simulink model "BrowarModel"  (R2024a)
settings: Solver=ode5  StartTime=0.0  StopTime=inf  FixedStep=0.1  RelTol=1e-3
undefined symbols (not defined in the file or in its folder): localhost, Matrikon, OI
libraries: opclib x24
(part 9 of 9)

== system BrowarModel/Mlyn browarniany/Mlyn browarniany/Zasobnik dozownika slodu/Detektory poziomu ==
  note: Detektory poziomu
  Poziom : Inport
  Pozycja sensora max (5 m) : Constant  Value=5
  Pozycja sensora min (2 m) : Constant  Value=2
  Sensor max : RelationalOperator  InputSameDT=off
  Sensor min : RelationalOperator  InputSameDT=off
  Poziom  wysoki : Outport
  Poziom niski : Outport  Port=2
  wires:
  Sensor min/1 -> Poziom niski/1
  Sensor max/1 -> Poziom  wysoki/1
  Pozycja sensora min (2 m)/1 -> Sensor min/2
  Pozycja sensora max (5 m)/1 -> Sensor max/2
  Poziom/1 -> Sensor max/1, Sensor min/1  "m"

== system BrowarModel/Mlyn browarniany/Mlyn browarniany/Zawor doplywu slodu/Zaklocenia ==
  note: Zaklocenia procesowe
  In : Inport
  Product3 : Product  InputSameDT=on  RndMeth=Zero  SaturateOnIntegerOverflow=on  OutDataTypeStr=Inherit: Same as first input
  Product4 : Product  InputSameDT=on  RndMeth=Zero  SaturateOnIntegerOverflow=on  OutDataTypeStr=Inherit: Same as first input
  Random Number : RandomNumber  Variance=0.01  Seed=4365624  SampleTime=0.1
  Transfer Fcn1 : TransferFcn  Denominator=[0.1 1]
  Out : Outport
  wires:
  [ZaklProc] -> Product3/2
  Random Number/1 -> Product3/1
  Product3/1 -> Transfer Fcn1/1
  Transfer Fcn1/1 -> Product4/2
  In/1 -> Product4/1
  Product4/1 -> Out/1

== system BrowarModel/System dozowania chmielu/System dozowania chmielu/Zasobnik/Detektory poziomu ==
  note: Detektory poziomu
  Poziom : Inport
  Pozycja sensora max (3 m) : Constant  Value=3
  Pozycja sensora min (1 m) : Constant
  Sensor max : RelationalOperator  InputSameDT=off
  Sensor min : RelationalOperator  InputSameDT=off
  Poziom  wysoki : Outport
  Poziom niski : Outport  Port=2
  wires:
  Sensor min/1 -> Poziom niski/1
  Sensor max/1 -> Poziom  wysoki/1
  Pozycja sensora min (1 m)/1 -> Sensor min/2
  Pozycja sensora max (3 m)/1 -> Sensor max/2
  Poziom/1 -> Sensor max/1, Sensor min/1  "m"

== system BrowarModel/System dozowania chmielu/System dozowania chmielu/Zawor doplywu chmielu/Zaklocenia ==
  note: Zaklocenia procesowe
  In : Inport
  Product3 : Product  InputSameDT=on  RndMeth=Zero  SaturateOnIntegerOverflow=on  OutDataTypeStr=Inherit: Same as first input
  Product4 : Product  InputSameDT=on  RndMeth=Zero  SaturateOnIntegerOverflow=on  OutDataTypeStr=Inherit: Same as first input
  Random Number : RandomNumber  Variance=0.01  Seed=4365624  SampleTime=0.1
  Transfer Fcn1 : TransferFcn  Denominator=[0.1 1]
  Out : Outport
  wires:
  [ZaklProc] -> Product3/2
  Random Number/1 -> Product3/1
  Product3/1 -> Transfer Fcn1/1
  Transfer Fcn1/1 -> Product4/2
  In/1 -> Product4/1
  Product4/1 -> Out/1

== system BrowarModel/System dozowania drozdzy/System dozowania drozdzy/Zasobnik/Detektory poziomu ==
  note: Detektory poziomu
  Poziom : Inport
  Pozycja sensora max (3 m) : Constant  Value=3
  Pozycja sensora min (1 m) : Constant
  Sensor max : RelationalOperator  InputSameDT=off
  Sensor min : RelationalOperator  InputSameDT=off
  Poziom  wysoki : Outport
  Poziom niski : Outport  Port=2
  wires:
  Sensor min/1 -> Poziom niski/1
  Sensor max/1 -> Poziom  wysoki/1
  Pozycja sensora min (1 m)/1 -> Sensor min/2
  Pozycja sensora max (3 m)/1 -> Sensor max/2
  Poziom/1 -> Sensor max/1, Sensor min/1  "m"

== system BrowarModel/System dozowania drozdzy/System dozowania drozdzy/Zawor doplywu drozdzy/Zaklocenia ==
  note: Zaklocenia procesowe
  In : Inport
  Product3 : Product  InputSameDT=on  RndMeth=Zero  SaturateOnIntegerOverflow=on  OutDataTypeStr=Inherit: Same as first input
  Product4 : Product  InputSameDT=on  RndMeth=Zero  SaturateOnIntegerOverflow=on  OutDataTypeStr=Inherit: Same as first input
  Random Number : RandomNumber  Variance=0.01  Seed=4365624  SampleTime=0.1
  Transfer Fcn1 : TransferFcn  Denominator=[0.1 1]
  Out : Outport
  wires:
  [ZaklProc] -> Product3/2
  Random Number/1 -> Product3/1
  Product3/1 -> Transfer Fcn1/1
  Transfer Fcn1/1 -> Product4/2
  In/1 -> Product4/1
  Product4/1 -> Out/1

== system BrowarModel/Kadz fermentacyjna/Kadz fermentacyjna/Kadz/Model akumulacji ciepla w zbiorniku z ciecza/Cieplo strumienia cieczy doplywajacej ==
  Temperatura strumienia cieczy : Inport
  Strumien cieczy : Inport  Port=2
  "  Dot " : DotProduct  OutDataTypeStr=Inherit: Inherit via internal rule
  Cieplo wlasciwe : Constant  Value=4189.9
  Dot : DotProduct  OutDataTypeStr=Inherit: Inherit via internal rule
  Gestosc cieczy : Gain  Gain=1000
  Sum9 : Sum  Inputs=|++
  "Zamiana C->K " : Constant  Value=273.6
  Strumien ciepla : Outport
  wires:
  Cieplo wlasciwe/1 -> Dot/1  "J/(kg*K)"
  Sum9/1 -> Dot/2  "dec K"
  "Zamiana C->K "/1 -> Sum9/2
  Dot/1 -> "  Dot "/1
  Gestosc cieczy/1 -> "  Dot "/2  "kg/s"
  Temperatura strumienia cieczy/1 -> Sum9/1
  "  Dot "/1 -> Strumien ciepla/1  "J/s"
  Strumien cieczy/1 -> Gestosc cieczy/1

== system BrowarModel/Kadz fermentacyjna/Kadz fermentacyjna/Kadz/Model akumulacji ciepla w zbiorniku z ciecza/Cieplo strumienia cieczy odplywajacej ==
  Temperatura strumienia cieczy : Inport
  Strumien cieczy : Inport  Port=2
  " Dot " : DotProduct  OutDataTypeStr=Inherit: Inherit via internal rule
  Cieplo wlasciwe : Constant  Value=4189.9
  "Dot " : DotProduct  OutDataTypeStr=Inherit: Inherit via internal rule
  Gestosc : Gain  Gain=1000
  Strumien ciepla : Outport
  wires:
  "Dot "/1 -> " Dot "/2
  Cieplo wlasciwe/1 -> "Dot "/2  "J/(kg*K)"
  Temperatura strumienia cieczy/1 -> " Dot "/1  "decK"
  Strumien cieczy/1 -> Gestosc/1  "m3/s"
  " Dot "/1 -> Strumien ciepla/1  "J/s"
  Gestosc/1 -> "Dot "/1  "kg/s"

== system BrowarModel/Kadz fermentacyjna/Kadz fermentacyjna/Kadz/Model rozkladu temperatur/Model rozkladu temperatur ==
  Poziom : Inport
  Temperatura otoczenia : Inport  Port=2
  Srednia temperatura : Inport  Port=3
  Obroty mieszadla : Inport  Port=4
  "  1/2  " : Gain  Gain=0.5
  " Dot  1" : DotProduct  OutDataTypeStr=Inherit: Inherit via internal rule
  " Gain 2" : Gain  Gain=2
  "1/2  " : Gain  Gain=0.5
  Fcn : Fcn  Expr=0.9*u(1)*(1-0.9*u(2))
  MinMax : MinMax
  Mux : Mux  Inputs=2
  Mux1 : Mux  Inputs=2
  Obroty skalowanie : Gain  Gain=1/2
  Poziom FS1 : Gain  Gain=1/2
  Sat : Saturate  UpperLimit=100  LowerLimit=0
  Sat doplyw Sat FS : Saturate  UpperLimit=1  LowerLimit=0
  Sat doplyw Sat FS1 : Saturate  UpperLimit=1  LowerLimit=0
  Saturation : Saturate  UpperLimit=100  LowerLimit=0
  Saturation1 : Saturate  UpperLimit=100  LowerLimit=0
  Sum1 : Sum  Inputs=|++
  Sum2 : Sum  Inputs=|-+
  Sum3 : Sum  Inputs=|+-
  Sum4 : Sum  Inputs=|-+
  Sum5 : Sum  Inputs=|++
  Sum7 : Sum  Inputs=|-+
  Sum8 : Sum  Inputs=|++
  Transfer Fcn : TransferFcn  Denominator=[10 1]
  Temperatura przy powierzchni : Outport
  Temperatura przy dnie : Outport  Port=2
  Gradient temperatury : Outport  Port=3
  wires:
  Srednia temperatura/1 -> Sum8/2, Sum4/2, Sum1/2, Sum2/2, Sum3/2, Sum5/2, Sum7/2
  Transfer Fcn/1 -> Sat doplyw Sat FS1/1
  Sat doplyw Sat FS1/1 -> " Dot  1"/1
  Sum4/1 -> " Dot  1"/2
  " Dot  1"/1 -> "1/2  "/1, "  1/2  "/1
  "1/2  "/1 -> Sum1/1
  "  1/2  "/1 -> Sum2/1
  Sum2/1 -> Saturation/1
  Sum1/1 -> Saturation1/1
  Saturation1/1 -> Sum3/1
  Saturation/1 -> Sum5/1
  Sum5/1 -> Mux/1
  Sum3/1 -> Mux/2
  Mux/1 -> MinMax/1
  MinMax/1 -> Sat/1
  Sat/1 -> Sum8/1, Sum7/1, " Gain 2"/1
  Temperatura otoczenia/1 -> Sum4/1
  Sum7/1 -> Temperatura przy powierzchni/1
  " Gain 2"/1 -> Gradient temperatury/1
  Sum8/1 -> Temperatura przy dnie/1
  Mux1/1 -> Fcn/1
  Poziom FS1/1 -> Mux1/1
  Sat doplyw Sat FS/1 -> Mux1/2
  Poziom/1 -> Poziom FS1/1  "m"
  Obroty mieszadla/1 -> Obroty skalowanie/1  "obr/min"
  Obroty skalowanie/1 -> Sat doplyw Sat FS/1  "FS"
  Fcn/1 -> Transfer Fcn/1

== system BrowarModel/Kadz fermentacyjna/Kadz fermentacyjna/Odplyw z kadzi/Silnik elektryczny/Stan ==
  Zalaczony : Inport
  Zdatny : Inport  Port=2
  Add : Sum  Inputs=+++
  Alarm1 : Logic  Operator=NOT  AllPortsSameDT=off
  Alarm2 : Gain  Gain=3
  Display : Display
  GUIMon : Gain
  Idle1 : Logic  AllPortsSameDT=off
  Idle2 : Logic  Operator=NOT  AllPortsSameDT=off
  Idle3 : Gain
  Running1 : Logic  AllPortsSameDT=off
  Running2 : Gain  Gain=2
  Idle : Outport
  Running : Outport  Port=2
  Alarm : Outport  Port=3
  wires:
  Running1/1 -> Running/1, Running2/1
  Idle1/1 -> Idle/1, Idle3/1
  Zalaczony/1 -> Running1/1, Idle2/1
  Zdatny/1 -> Alarm1/1, Running1/2, Idle1/2
  Alarm1/1 -> Alarm/1, Alarm2/1
  Idle2/1 -> Idle1/1
  Idle3/1 -> Add/1
  Running2/1 -> Add/2
  Alarm2/1 -> Add/3
  Add/1 -> GUIMon/1
  GUIMon/1 -> Display/1

== system BrowarModel/Kadz fermentacyjna/Kadz fermentacyjna/Odplyw z kadzi/Silnik elektryczny/Sterowanie ==
  note: Sterowanie silnika elektrycznego
  Zadane obroty : Inport
  Zalaczenie : Inport  Port=2
  Hz : Gain  Gain=45/100
  Min sterowanie : Constant  Value=5
  Relay : Relay
  Saturation [0,100] : Saturate  UpperLimit=100  LowerLimit=0
  "Sterowanie " : DotProduct  OutDataTypeStr=Inherit: Inherit via internal rule
  Sum2 : Sum  Inputs=|++
  Sterowanie : Outport
  wires:
  Relay/1 -> "Sterowanie "/1  "{0,1}"
  Saturation [0,100]/1 -> Hz/1
  Hz/1 -> Sum2/1  "Hz"
  Min sterowanie/1 -> Sum2/2  "Hz"
  Sum2/1 -> "Sterowanie "/2
  Zalaczenie/1 -> Relay/1  "{0,1}"
  "Sterowanie "/1 -> Sterowanie/1  "Hz"
  Zadane obroty/1 -> Saturation [0,100]/1  "[0,100]"

== system BrowarModel/Kadz fermentacyjna/Kadz fermentacyjna/Odplyw z kadzi/Silnik elektryczny/Sterownik ==
  PV : Inport
  SP : Inport  Port=2
  Integrator : Integrator  LimitOutput=on  UpperSaturationLimit=50  LowerSaturationLimit=0
  K : Gain
  Saturation [0,50] : Saturate  UpperLimit=50  LowerLimit=0
  Sum2 : Sum  Inputs=|+-
  Sum3 : Sum  Inputs=|++
  Ti : Gain
  CV : Outport
  wires:
  Sum2/1 -> K/1
  Integrator/1 -> Sum3/1
  K/1 -> Ti/1, Sum3/2
  Ti/1 -> Integrator/1
  PV/1 -> Sum2/2
  SP/1 -> Sum2/1
  Sum3/1 -> Saturation [0,50]/1
  Saturation [0,50]/1 -> CV/1

== system BrowarModel/Kadz fermentacyjna/Kadz fermentacyjna/Odplyw z kadzi/Silnik elektryczny/Zaklocenia ==
  note: Zaklocenia procesowe
  In : Inport
  Product3 : Product  InputSameDT=on  RndMeth=Zero  SaturateOnIntegerOverflow=on  OutDataTypeStr=Inherit: Same as first input
  Product4 : Product  InputSameDT=on  RndMeth=Zero  SaturateOnIntegerOverflow=on  OutDataTypeStr=Inherit: Same as first input
  Random Number : RandomNumber  Variance=0.05  Seed=4365624  SampleTime=0.1
  Transfer Fcn1 : TransferFcn  Denominator=[1 1]
  Transfer Fcn2 : TransferFcn  Denominator=[1 1]
  Transfer Fcn3 : TransferFcn  Denominator=[1 1]
  Out : Outport
  wires:
  [ZaklProc] -> Product3/2
  Random Number/1 -> Product3/1
  Product3/1 -> Transfer Fcn1/1
  Transfer Fcn1/1 -> Transfer Fcn2/1
  In/1 -> Product4/1
  Product4/1 -> Out/1
  Transfer Fcn2/1 -> Transfer Fcn3/1
  Transfer Fcn3/1 -> Product4/2

== system BrowarModel/Kadz filtracji/Kadz filtracji/Doplyw kadzi/Silnik elektryczny/Stan ==
  Zalaczony : Inport
  Zdatny : Inport  Port=2
  Add : Sum  Inputs=+++
  Alarm1 : Logic  Operator=NOT  AllPortsSameDT=off
  Alarm2 : Gain  Gain=3
  Display : Display
  GUIMon : Gain
  Idle1 : Logic  AllPortsSameDT=off
  Idle2 : Logic  Operator=NOT  AllPortsSameDT=off
  Idle3 : Gain
  Running1 : Logic  AllPortsSameDT=off
  Running2 : Gain  Gain=2
  Idle : Outport
  Running : Outport  Port=2
  Alarm : Outport  Port=3
  wires:
  Running1/1 -> Running/1, Running2/1
  Idle1/1 -> Idle/1, Idle3/1
  Zalaczony/1 -> Running1/1, Idle2/1
  Zdatny/1 -> Alarm1/1, Running1/2, Idle1/2
  Alarm1/1 -> Alarm/1, Alarm2/1
  Idle2/1 -> Idle1/1
  Idle3/1 -> Add/1
  Running2/1 -> Add/2
  Alarm2/1 -> Add/3
  Add/1 -> GUIMon/1
  GUIMon/1 -> Display/1

== system BrowarModel/Kadz filtracji/Kadz filtracji/Doplyw kadzi/Silnik elektryczny/Sterowanie ==
  note: Sterowanie silnika elektrycznego
  Zadane obroty : Inport
  Zalaczenie : Inport  Port=2
  Hz : Gain  Gain=45/100
  Min sterowanie : Constant  Value=5
  Relay : Relay
  Saturation [0,100] : Saturate  UpperLimit=100  LowerLimit=0
  "Sterowanie " : DotProduct  OutDataTypeStr=Inherit: Inherit via internal rule
  Sum2 : Sum  Inputs=|++
  Sterowanie : Outport
  wires:
  Relay/1 -> "Sterowanie "/1  "{0,1}"
  Saturation [0,100]/1 -> Hz/1
  Hz/1 -> Sum2/1  "Hz"
  Min sterowanie/1 -> Sum2/2  "Hz"
  Sum2/1 -> "Sterowanie "/2
  Zalaczenie/1 -> Relay/1  "{0,1}"
  "Sterowanie "/1 -> Sterowanie/1  "Hz"
  Zadane obroty/1 -> Saturation [0,100]/1  "[0,100]"

== system BrowarModel/Kadz filtracji/Kadz filtracji/Doplyw kadzi/Silnik elektryczny/Sterownik ==
  PV : Inport
  SP : Inport  Port=2
  Integrator : Integrator  LimitOutput=on  UpperSaturationLimit=50  LowerSaturationLimit=0
  K : Gain
  Saturation [0,50] : Saturate  UpperLimit=50  LowerLimit=0
  Sum2 : Sum  Inputs=|+-
  Sum3 : Sum  Inputs=|++
  Ti : Gain
  CV : Outport
  wires:
  Sum2/1 -> K/1
  Integrator/1 -> Sum3/1
  K/1 -> Ti/1, Sum3/2
  Ti/1 -> Integrator/1
  PV/1 -> Sum2/2
  SP/1 -> Sum2/1
  Sum3/1 -> Saturation [0,50]/1
  Saturation [0,50]/1 -> CV/1

== system BrowarModel/Kadz filtracji/Kadz filtracji/Doplyw kadzi/Silnik elektryczny/Zaklocenia ==
  note: Zaklocenia procesowe
  In : Inport
  Product3 : Product  InputSameDT=on  RndMeth=Zero  SaturateOnIntegerOverflow=on  OutDataTypeStr=Inherit: Same as first input
  Product4 : Product  InputSameDT=on  RndMeth=Zero  SaturateOnIntegerOverflow=on  OutDataTypeStr=Inherit: Same as first input
  Random Number : RandomNumber  Variance=0.05  Seed=4365624  SampleTime=0.1
  Transfer Fcn1 : TransferFcn  Denominator=[1 1]
  Transfer Fcn2 : TransferFcn  Denominator=[1 1]
  Transfer Fcn3 : TransferFcn  Denominator=[1 1]
  Out : Outport
  wires:
  [ZaklProc] -> Product3/2
  Random Number/1 -> Product3/1
  Product3/1 -> Transfer Fcn1/1
  Transfer Fcn1/1 -> Transfer Fcn2/1
  In/1 -> Product4/1
  Product4/1 -> Out/1
  Transfer Fcn2/1 -> Transfer Fcn3/1
  Transfer Fcn3/1 -> Product4/2

== system BrowarModel/Kadz filtracji/Kadz filtracji/Odplyw + cyrkulacja/Silnik elektryczny/Stan ==
  Zalaczony : Inport
  Zdatny : Inport  Port=2
  Add : Sum  Inputs=+++
  Alarm1 : Logic  Operator=NOT  AllPortsSameDT=off
  Alarm2 : Gain  Gain=3
  Display : Display
  GUIMon : Gain
  Idle1 : Logic  AllPortsSameDT=off
  Idle2 : Logic  Operator=NOT  AllPortsSameDT=off
  Idle3 : Gain
  Running1 : Logic  AllPortsSameDT=off
  Running2 : Gain  Gain=2
  Idle : Outport
  Running : Outport  Port=2
  Alarm : Outport  Port=3
  wires:
  Running1/1 -> Running/1, Running2/1
  Idle1/1 -> Idle/1, Idle3/1
  Zalaczony/1 -> Running1/1, Idle2/1
  Zdatny/1 -> Alarm1/1, Running1/2, Idle1/2
  Alarm1/1 -> Alarm/1, Alarm2/1
  Idle2/1 -> Idle1/1
  Idle3/1 -> Add/1
  Running2/1 -> Add/2
  Alarm2/1 -> Add/3
  Add/1 -> GUIMon/1
  GUIMon/1 -> Display/1

== system BrowarModel/Kadz filtracji/Kadz filtracji/Odplyw + cyrkulacja/Silnik elektryczny/Sterowanie ==
  note: Sterowanie silnika elektrycznego
  Zadane obroty : Inport
  Zalaczenie : Inport  Port=2
  Hz : Gain  Gain=45/100
  Min sterowanie : Constant  Value=5
  Relay : Relay
  Saturation [0,100] : Saturate  UpperLimit=100  LowerLimit=0
  "Sterowanie " : DotProduct  OutDataTypeStr=Inherit: Inherit via internal rule
  Sum2 : Sum  Inputs=|++
  Sterowanie : Outport
  wires:
  Relay/1 -> "Sterowanie "/1  "{0,1}"
  Saturation [0,100]/1 -> Hz/1
  Hz/1 -> Sum2/1  "Hz"
  Min sterowanie/1 -> Sum2/2  "Hz"
  Sum2/1 -> "Sterowanie "/2
  Zalaczenie/1 -> Relay/1  "{0,1}"
  "Sterowanie "/1 -> Sterowanie/1  "Hz"
  Zadane obroty/1 -> Saturation [0,100]/1  "[0,100]"

== system BrowarModel/Kadz filtracji/Kadz filtracji/Odplyw + cyrkulacja/Silnik elektryczny/Sterownik ==
  PV : Inport
  SP : Inport  Port=2
  Integrator : Integrator  LimitOutput=on  UpperSaturationLimit=50  LowerSaturationLimit=0
  K : Gain
  Saturation [0,50] : Saturate  UpperLimit=50  LowerLimit=0
  Sum2 : Sum  Inputs=|+-
  Sum3 : Sum  Inputs=|++
  Ti : Gain
  CV : Outport
  wires:
  Sum2/1 -> K/1
  Integrator/1 -> Sum3/1
  K/1 -> Ti/1, Sum3/2
  Ti/1 -> Integrator/1
  PV/1 -> Sum2/2
  SP/1 -> Sum2/1
  Sum3/1 -> Saturation [0,50]/1
  Saturation [0,50]/1 -> CV/1

== system BrowarModel/Kadz filtracji/Kadz filtracji/Odplyw + cyrkulacja/Silnik elektryczny/Zaklocenia ==
  note: Zaklocenia procesowe
  In : Inport
  Product3 : Product  InputSameDT=on  RndMeth=Zero  SaturateOnIntegerOverflow=on  OutDataTypeStr=Inherit: Same as first input
  Product4 : Product  InputSameDT=on  RndMeth=Zero  SaturateOnIntegerOverflow=on  OutDataTypeStr=Inherit: Same as first input
  Random Number : RandomNumber  Variance=0.05  Seed=4365624  SampleTime=0.1
  Transfer Fcn1 : TransferFcn  Denominator=[1 1]
  Transfer Fcn2 : TransferFcn  Denominator=[1 1]
  Transfer Fcn3 : TransferFcn  Denominator=[1 1]
  Out : Outport
  wires:
  [ZaklProc] -> Product3/2
  Random Number/1 -> Product3/1
  Product3/1 -> Transfer Fcn1/1
  Transfer Fcn1/1 -> Transfer Fcn2/1
  In/1 -> Product4/1
  Product4/1 -> Out/1
  Transfer Fcn2/1 -> Transfer Fcn3/1
  Transfer Fcn3/1 -> Product4/2

== system BrowarModel/Kadz filtracji/Kadz filtracji/Zbiornik dolny/Model akumulacji ciepla w zbiorniku/Cieplo strumienia cieczy odplywajacej ==
  note: Cieplo strumienia cieczy odplywajacej
  Temperatura strumienia cieczy : Inport
  Strumien cieczy : Inport  Port=2
  " Dot " : DotProduct  OutDataTypeStr=Inherit: Inherit via internal rule
  Cieplo wlasciwe : Constant  Value=4189.9
  "Dot " : DotProduct  OutDataTypeStr=Inherit: Inherit via internal rule
  Gestosc : Gain  Gain=1000
  Strumien ciepla : Outport
  wires:
  Gestosc/1 -> "Dot "/1  "kg/s"
  " Dot "/1 -> Strumien ciepla/1  "J/s"
  Strumien cieczy/1 -> Gestosc/1  "m3/s"
  Temperatura strumienia cieczy/1 -> " Dot "/1  "decK"
  Cieplo wlasciwe/1 -> "Dot "/2  "J/(kg*K)"
  "Dot "/1 -> " Dot "/2

== system BrowarModel/Kadz filtracji/Kadz filtracji/Zbiornik dolny/Model akumulacji ciepla w zbiorniku/Cieplo strumienia doplywajacego ==
  note: Cieplo strumienia doplywajacego
  Temperatura strumienia brzeczki : Inport
  Strumien brzeczki : Inport  Port=2
  "  Dot  " : DotProduct  OutDataTypeStr=Inherit: Inherit via internal rule
  Cieplo wlasciwe brzeczki : Constant  Value=4189.9
  "Dot  " : DotProduct  OutDataTypeStr=Inherit: Inherit via internal rule
  Gestosc brzeczki : Gain  Gain=1000
  Sum3 : Sum  Inputs=|++
  "Zamiana C->K  " : Constant  Value=273.6
  Strumien ciepla : Outport
  wires:
  Strumien brzeczki/1 -> Gestosc brzeczki/1
  Temperatura strumienia brzeczki/1 -> Sum3/1
  Gestosc brzeczki/1 -> "  Dot  "/2  "kg/s"
  "Dot  "/1 -> "  Dot  "/1
  "Zamiana C->K  "/1 -> Sum3/2
  Sum3/1 -> "Dot  "/2  "dec K"
  Cieplo wlasciwe brzeczki/1 -> "Dot  "/1  "J/(kg*K)"
  "  Dot  "/1 -> Strumien ciepla/1  "J/s"

== system BrowarModel/Kadz filtracji/Kadz filtracji/Zbiornik gorny/Model akumulacji ciepla w zbiorniku/Cieplo strumienia cieczy odplywajacej ==
  note: Cieplo strumienia cieczy odplywajacej
  Temperatura strumienia cieczy : Inport
  Strumien cieczy : Inport  Port=2
  " Dot " : DotProduct  OutDataTypeStr=Inherit: Inherit via internal rule
  Cieplo wlasciwe : Constant  Value=4189.9
  "Dot " : DotProduct  OutDataTypeStr=Inherit: Inherit via internal rule
  Gestosc : Gain  Gain=1000
  Strumien ciepla : Outport
  wires:
  Gestosc/1 -> "Dot "/1  "kg/s"
  " Dot "/1 -> Strumien ciepla/1  "J/s"
  Strumien cieczy/1 -> Gestosc/1  "m3/s"
  Temperatura strumienia cieczy/1 -> " Dot "/1  "decK"
  Cieplo wlasciwe/1 -> "Dot "/2  "J/(kg*K)"
  "Dot "/1 -> " Dot "/2

== system BrowarModel/Kadz filtracji/Kadz filtracji/Zbiornik gorny/Model akumulacji ciepla w zbiorniku/Cieplo strumienia doplywajacego ==
  note: Cieplo strumienia doplywajacego
  Temperatura strumienia wody : Inport
  Strumien wody : Inport  Port=2
  Temperatura strumienia zacieru : Inport  Port=3
  Strumien zacieru : Inport  Port=4
  Temperatura strumienia brzeczki : Inport  Port=5
  Strumien brzeczki : Inport  Port=6
  "  Dot " : DotProduct  OutDataTypeStr=Inherit: Inherit via internal rule
  "  Dot 1" : DotProduct  OutDataTypeStr=Inherit: Inherit via internal rule
  "  Dot 2" : DotProduct  OutDataTypeStr=Inherit: Inherit via internal rule
  Cieplo wlasciwe brzeczki : Constant  Value=4189.9
  Cieplo wlasciwe wody : Constant  Value=4189.9
  Cieplo wlasciwe zacieru : Constant  Value=4189.9
  Dot : DotProduct  OutDataTypeStr=Inherit: Inherit via internal rule
  Dot1 : DotProduct  OutDataTypeStr=Inherit: Inherit via internal rule
  Dot2 : DotProduct  OutDataTypeStr=Inherit: Inherit via internal rule
  Gestosc brzeczki : Gain  Gain=1000
  Gestosc wody : Gain  Gain=1000
  Gestosc zacieru : Gain  Gain=1000
  Sum{1..4,9} (5 alike) : Sum  Inputs=|++
  "Zamiana C->K " : Constant  Value=273.6
  "Zamiana C->K  " : Constant  Value=273.6
  Zamiana C->K 1 : Constant  Value=273.6
  Strumien ciepla : Outport
  wires:
  Strumien wody/1 -> Gestosc wody/1
  Temperatura strumienia wody/1 -> Sum9/1
  Gestosc wody/1 -> "  Dot "/2  "kg/s"
  Dot/1 -> "  Dot "/1
  "Zamiana C->K "/1 -> Sum9/2
  Sum9/1 -> Dot/2  "dec K"
  Cieplo wlasciwe wody/1 -> Dot/1  "J/(kg*K)"
  "  Dot "/1 -> Sum1/1  "J/s"
  Sum1/1 -> Strumien ciepla/1  "J/s"
  Strumien zacieru/1 -> Gestosc zacieru/1
  Temperatura strumienia zacieru/1 -> Sum2/1
  Gestosc zacieru/1 -> "  Dot 1"/2  "kg/s"
  Dot1/1 -> "  Dot 1"/1
  Zamiana C->K 1/1 -> Sum2/2
  Sum2/1 -> Dot1/2  "dec K"
  Cieplo wlasciwe zacieru/1 -> Dot1/1  "J/(kg*K)"
  Strumien brzeczki/1 -> Gestosc brzeczki/1
  Temperatura strumienia brzeczki/1 -> Sum3/1
  Gestosc brzeczki/1 -> "  Dot 2"/2  "kg/s"
  Dot2/1 -> "  Dot 2"/1
  "Zamiana C->K  "/1 -> Sum3/2
  Sum3/1 -> Dot2/2  "dec K"
  Cieplo wlasciwe brzeczki/1 -> Dot2/1  "J/(kg*K)"
  "  Dot 1"/1 -> Sum4/1  "J/s"
  Sum4/1 -> Sum1/2
  "  Dot 2"/1 -> Sum4/2  "J/s"

== system BrowarModel/Kadz filtracji/Kadz filtracji/Zbiornik gorny/Model filtru/Booster block ==
  Fast : Constant  Value=2
  Normal : Constant
  Switch : Switch  Threshold=0.5  SaturateOnIntegerOverflow=off  InputSameDT=off
  Out : Outport
  wires:
  [TrybSym] -> Switch/2
  Fast/1 -> Switch/1
  Normal/1 -> Switch/3
  Switch/1 -> Out/1

== system BrowarModel/Kadz filtracji/Kadz filtracji/Zbiornik gorny/Silnik elektryczny/Stan ==
  Zalaczony : Inport
  Zdatny : Inport  Port=2
  Add : Sum  Inputs=+++
  Alarm1 : Logic  Operator=NOT  AllPortsSameDT=off
  Alarm2 : Gain  Gain=3
  Display : Display
  GUIMon : Gain
  Idle1 : Logic  AllPortsSameDT=off
  Idle2 : Logic  Operator=NOT  AllPortsSameDT=off
  Idle3 : Gain
  Running1 : Logic  AllPortsSameDT=off
  Running2 : Gain  Gain=2
  Idle : Outport
  Running : Outport  Port=2
  Alarm : Outport  Port=3
  wires:
  Running1/1 -> Running/1, Running2/1
  Idle1/1 -> Idle/1, Idle3/1
  Zalaczony/1 -> Running1/1, Idle2/1
  Zdatny/1 -> Alarm1/1, Running1/2, Idle1/2
  Alarm1/1 -> Alarm/1, Alarm2/1
  Idle2/1 -> Idle1/1
  Idle3/1 -> Add/1
  Running2/1 -> Add/2
  Alarm2/1 -> Add/3
  Add/1 -> GUIMon/1
  GUIMon/1 -> Display/1

== system BrowarModel/Kadz filtracji/Kadz filtracji/Zbiornik gorny/Silnik elektryczny/Sterowanie ==
  note: Sterowanie silnika elektrycznego
  Zadane obroty : Inport
  Zalaczenie : Inport  Port=2
  Hz : Gain  Gain=45/100
  Min sterowanie : Constant  Value=5
  Relay : Relay
  Saturation [0,100] : Saturate  UpperLimit=100  LowerLimit=0
  "Sterowanie " : DotProduct  OutDataTypeStr=Inherit: Inherit via internal rule
  Sum2 : Sum  Inputs=|++
  Sterowanie : Outport
  wires:
  Relay/1 -> "Sterowanie "/1  "{0,1}"
  Saturation [0,100]/1 -> Hz/1
  Hz/1 -> Sum2/1  "Hz"
  Min sterowanie/1 -> Sum2/2  "Hz"
  Sum2/1 -> "Sterowanie "/2
  Zalaczenie/1 -> Relay/1  "{0,1}"
  "Sterowanie "/1 -> Sterowanie/1  "Hz"
  Zadane obroty/1 -> Saturation [0,100]/1  "[0,100]"

== system BrowarModel/Kadz filtracji/Kadz filtracji/Zbiornik gorny/Silnik elektryczny/Sterownik ==
  PV : Inport
  SP : Inport  Port=2
  Integrator : Integrator  LimitOutput=on  UpperSaturationLimit=50  LowerSaturationLimit=0
  K : Gain
  Saturation [0,50] : Saturate  UpperLimit=50  LowerLimit=0
  Sum2 : Sum  Inputs=|+-
  Sum3 : Sum  Inputs=|++
  Ti : Gain
  CV : Outport
  wires:
  Sum2/1 -> K/1
  Integrator/1 -> Sum3/1
  K/1 -> Ti/1, Sum3/2
  Ti/1 -> Integrator/1
  PV/1 -> Sum2/2
  SP/1 -> Sum2/1
  Sum3/1 -> Saturation [0,50]/1
  Saturation [0,50]/1 -> CV/1

== system BrowarModel/Kadz filtracji/Kadz filtracji/Zbiornik gorny/Silnik elektryczny/Zaklocenia ==
  note: Zaklocenia procesowe
  In : Inport
  Product3 : Product  InputSameDT=on  RndMeth=Zero  SaturateOnIntegerOverflow=on  OutDataTypeStr=Inherit: Same as first input
  Product4 : Product  InputSameDT=on  RndMeth=Zero  SaturateOnIntegerOverflow=on  OutDataTypeStr=Inherit: Same as first input
  Random Number : RandomNumber  Variance=0.05  Seed=4365624  SampleTime=0.1
  Transfer Fcn1 : TransferFcn  Denominator=[1 1]
  Transfer Fcn2 : TransferFcn  Denominator=[1 1]
  Transfer Fcn3 : TransferFcn  Denominator=[1 1]
  Out : Outport
  wires:
  [ZaklProc] -> Product3/2
  Random Number/1 -> Product3/1
  Product3/1 -> Transfer Fcn1/1
  Transfer Fcn1/1 -> Transfer Fcn2/1
  In/1 -> Product4/1
  Product4/1 -> Out/1
  Transfer Fcn2/1 -> Transfer Fcn3/1
  Transfer Fcn3/1 -> Product4/2

== system BrowarModel/Kadz warzelna/Kadz warzelna/Model jakosci warzenia/Gotowanie /Booster block ==
  Fast : Constant  Value=12
  Normal : Constant
  Switch : Switch  Threshold=0.5  SaturateOnIntegerOverflow=off  InputSameDT=off
  Out : Outport
  wires:
  [TrybSym] -> Switch/2
  Fast/1 -> Switch/1
  Normal/1 -> Switch/3
  Switch/1 -> Out/1

== system BrowarModel/Kadz warzelna/Kadz warzelna/Odplyw z kadzi/Silnik elektryczny/Stan ==
  Zalaczony : Inport
  Zdatny : Inport  Port=2
  Add : Sum  Inputs=+++
  Alarm1 : Logic  Operator=NOT  AllPortsSameDT=off
  Alarm2 : Gain  Gain=3
  Display : Display
  GUIMon : Gain
  Idle1 : Logic  AllPortsSameDT=off
  Idle2 : Logic  Operator=NOT  AllPortsSameDT=off
  Idle3 : Gain
  Running1 : Logic  AllPortsSameDT=off
  Running2 : Gain  Gain=2
  Idle : Outport
  Running : Outport  Port=2
  Alarm : Outport  Port=3
  wires:
  Running1/1 -> Running/1, Running2/1
  Idle1/1 -> Idle/1, Idle3/1
  Zalaczony/1 -> Running1/1, Idle2/1
  Zdatny/1 -> Alarm1/1, Running1/2, Idle1/2
  Alarm1/1 -> Alarm/1, Alarm2/1
  Idle2/1 -> Idle1/1
  Idle3/1 -> Add/1
  Running2/1 -> Add/2
  Alarm2/1 -> Add/3
  Add/1 -> GUIMon/1
  GUIMon/1 -> Display/1

== system BrowarModel/Kadz warzelna/Kadz warzelna/Odplyw z kadzi/Silnik elektryczny/Sterowanie ==
  note: Sterowanie silnika elektrycznego
  Zadane obroty : Inport
  Zalaczenie : Inport  Port=2
  Hz : Gain  Gain=45/100
  Min sterowanie : Constant  Value=5
  Relay : Relay
  Saturation [0,100] : Saturate  UpperLimit=100  LowerLimit=0
  "Sterowanie " : DotProduct  OutDataTypeStr=Inherit: Inherit via internal rule
  Sum2 : Sum  Inputs=|++
  Sterowanie : Outport
  wires:
  Relay/1 -> "Sterowanie "/1  "{0,1}"
  Saturation [0,100]/1 -> Hz/1
  Hz/1 -> Sum2/1  "Hz"
  Min sterowanie/1 -> Sum2/2  "Hz"
  Sum2/1 -> "Sterowanie "/2
  Zalaczenie/1 -> Relay/1  "{0,1}"
  "Sterowanie "/1 -> Sterowanie/1  "Hz"
  Zadane obroty/1 -> Saturation [0,100]/1  "[0,100]"

== system BrowarModel/Kadz warzelna/Kadz warzelna/Odplyw z kadzi/Silnik elektryczny/Sterownik ==
  PV : Inport
  SP : Inport  Port=2
  Integrator : Integrator  LimitOutput=on  UpperSaturationLimit=50  LowerSaturationLimit=0
  K : Gain
  Saturation [0,50] : Saturate  UpperLimit=50  LowerLimit=0
  Sum2 : Sum  Inputs=|+-
  Sum3 : Sum  Inputs=|++
  Ti : Gain
  CV : Outport
  wires:
  Sum2/1 -> K/1
  Integrator/1 -> Sum3/1
  K/1 -> Ti/1, Sum3/2
  Ti/1 -> Integrator/1
  PV/1 -> Sum2/2
  SP/1 -> Sum2/1
  Sum3/1 -> Saturation [0,50]/1
  Saturation [0,50]/1 -> CV/1

== system BrowarModel/Kadz warzelna/Kadz warzelna/Odplyw z kadzi/Silnik elektryczny/Zaklocenia ==
  note: Zaklocenia procesowe
  In : Inport
  Product3 : Product  InputSameDT=on  RndMeth=Zero  SaturateOnIntegerOverflow=on  OutDataTypeStr=Inherit: Same as first input
  Product4 : Product  InputSameDT=on  RndMeth=Zero  SaturateOnIntegerOverflow=on  OutDataTypeStr=Inherit: Same as first input
  Random Number : RandomNumber  Variance=0.05  Seed=4365624  SampleTime=0.1
  Transfer Fcn1 : TransferFcn  Denominator=[1 1]
  Transfer Fcn2 : TransferFcn  Denominator=[1 1]
  Transfer Fcn3 : TransferFcn  Denominator=[1 1]
  Out : Outport
  wires:
  [ZaklProc] -> Product3/2
  Random Number/1 -> Product3/1
  Product3/1 -> Transfer Fcn1/1
  Transfer Fcn1/1 -> Transfer Fcn2/1
  In/1 -> Product4/1
  Product4/1 -> Out/1
  Transfer Fcn2/1 -> Transfer Fcn3/1
  Transfer Fcn3/1 -> Product4/2

== system BrowarModel/Kadz zacierna/Kadz zacierna/Kadz zacierna/Model akumulacji ciepla w zbiorniku z ciecza/Cieplo strumienia cieczy odplywajacej ==
  note: Cieplo strumienia cieczy odplywajacej
  Temperatura strumienia cieczy : Inport
  Strumien cieczy : Inport  Port=2
  " Dot " : DotProduct  OutDataTypeStr=Inherit: Inherit via internal rule
  Cieplo wlasciwe : Constant  Value=4189.9
  "Dot " : DotProduct  OutDataTypeStr=Inherit: Inherit via internal rule
  Gestosc : Gain  Gain=1000
  Strumien ciepla : Outport
  wires:
  Gestosc/1 -> "Dot "/1  "kg/s"
  " Dot "/1 -> Strumien ciepla/1  "J/s"
  Strumien cieczy/1 -> Gestosc/1  "m3/s"
  Temperatura strumienia cieczy/1 -> " Dot "/1  "decK"
  Cieplo wlasciwe/1 -> "Dot "/2  "J/(kg*K)"
  "Dot "/1 -> " Dot "/2

== system BrowarModel/Kadz zacierna/Kadz zacierna/Kadz zacierna/Model akumulacji ciepla w zbiorniku z ciecza/Cieplo strumienia doplywajacego ==
  note: Cieplo strumienia doplywajacego
  Temperatura strumienia wody : Inport
  Strumien wody : Inport  Port=2
  Temperatura strumienia sruty : Inport  Port=3
  Strumien sruty : Inport  Port=4
  "  Dot " : DotProduct  OutDataTypeStr=Inherit: Inherit via internal rule
  "  Dot 1" : DotProduct  OutDataTypeStr=Inherit: Inherit via internal rule
  Cieplo wlasciwe sruty : Constant  Value=4189.9
  Cieplo wlasciwe wody : Constant  Value=4189.9
  Dot : DotProduct  OutDataTypeStr=Inherit: Inherit via internal rule
  Dot1 : DotProduct  OutDataTypeStr=Inherit: Inherit via internal rule
  Gestosc sruty : Gain  Gain=1000
  Gestosc wody : Gain  Gain=1000
  Sum1 : Sum  Inputs=|++
  Sum2 : Sum  Inputs=|++
  Sum9 : Sum  Inputs=|++
  "Zamiana C->K " : Constant  Value=273.6
  Zamiana C->K 1 : Constant  Value=273.6
  Strumien ciepla : Outport
  wires:
  Strumien wody/1 -> Gestosc wody/1
  Temperatura strumienia wody/1 -> Sum9/1
  Gestosc wody/1 -> "  Dot "/2  "kg/s"
  Dot/1 -> "  Dot "/1
  "Zamiana C->K "/1 -> Sum9/2
  Sum9/1 -> Dot/2  "dec K"
  Cieplo wlasciwe wody/1 -> Dot/1  "J/(kg*K)"
  "  Dot "/1 -> Sum1/1  "J/s"
  Sum1/1 -> Strumien ciepla/1  "J/s"
  Strumien sruty/1 -> Gestosc sruty/1
  Temperatura strumienia sruty/1 -> Sum2/1
  Gestosc sruty/1 -> "  Dot 1"/2  "kg/s"
  Dot1/1 -> "  Dot 1"/1
  Zamiana C->K 1/1 -> Sum2/2
  Sum2/1 -> Dot1/2  "dec K"
  Cieplo wlasciwe sruty/1 -> Dot1/1  "J/(kg*K)"
  "  Dot 1"/1 -> Sum1/2  "J/s"

== system BrowarModel/Kadz zacierna/Kadz zacierna/Kadz zacierna/Model jakosci zacieru/Przerwa bialkowa  ==
  note: Przerwa bialkowa
  Srednia temperatura : Inport
  Jakosc mieszaniny : Inport  Port=2
  Objetosc mieszaniny : Inport  Port=3
  Odplyw : Inport  Port=4
  Obroty mieszadla : Inport  Port=5
  Booster : Product  RndMeth=Zero
  Booster block : Subsystem
  Constant : Constant  Value=0.2
  Divide : Product  Inputs=*/
  Dynamika rozkladu : Gain  Gain=1/100
  Ilosc : Integrator  LimitOutput=on  UpperSaturationLimit=48  LowerSaturationLimit=0
  Mieszadlo : DotProduct  OutDataTypeStr=Inherit: Inherit via internal rule
  Nasycenie : DotProduct  OutDataTypeStr=Inherit: Inherit via internal rule
  Odplyw srutu : DotProduct  OutDataTypeStr=Inherit: Inherit via internal rule
  Relational Operator1 : RelationalOperator  Operator=>  InputSameDT=off
  Sum : Sum  Inputs=|++
  Sum8 : Sum  Inputs=|+-
  Sum9 : Sum  Inputs=|+-
  Szybkosc reakcji : DotProduct  OutDataTypeStr=Inherit: Inherit via internal rule
  Warunki rozkladu : DotProduct  OutDataTypeStr=Inherit: Inherit via internal rule
  Wplyw mpieszadla : Gain  Gain=0.8/0.9563
  Wplyw temperatury : Lookup  InputValues=[0, 46, 49, 50, 51, 54, 100]  Table=[0, 0, 1, 1, 1 0, 0]  SaturateOnIntegerOverflow=off
  Skrobia rozpuszczona : Outport
  wires:
  Wplyw temperatury/1 -> Warunki rozkladu/2
  Ilosc/1 -> Sum8/2, Divide/1
  Szybkosc reakcji/1 -> Nasycenie/2
  Divide/1 -> Odplyw srutu/2, Relational Operator1/2, Skrobia rozpuszczona/1
  Relational Operator1/1 -> Nasycenie/1
  Sum8/1 -> Szybkosc reakcji/2
  Sum9/1 -> Ilosc/1
  Nasycenie/1 -> Sum9/1
  Odplyw srutu/1 -> Sum9/2
  Srednia temperatura/1 -> Wplyw temperatury/1
  Objetosc mieszaniny/1 -> Divide/2, Sum8/1
  Odplyw/1 -> Odplyw srutu/1
  Jakosc mieszaniny/1 -> Warunki rozkladu/1, Relational Operator1/1
  Mieszadlo/1 -> Dynamika rozkladu/1
  Warunki rozkladu/1 -> Mieszadlo/2
  Obroty mieszadla/1 -> Wplyw mpieszadla/1
  Wplyw mpieszadla/1 -> Sum/1
  Constant/1 -> Sum/2
  Sum/1 -> Mieszadlo/1
  Booster block/1(Out) -> Booster/2
  Dynamika rozkladu/1 -> Booster/1
  Booster/1 -> Szybkosc reakcji/1

== system BrowarModel/Kadz zacierna/Kadz zacierna/Kadz zacierna/Model jakosci zacieru/Przerwa dekstrynujaca ==
  note: Przerwa dekstrynujaca
  Dekstryny : Inport
  Srednia temperatura : Inport  Port=2
  Jakosc mieszaniny : Inport  Port=3
  Objetosc mieszaniny : Inport  Port=4
  Odplyw : Inport  Port=5
  Obroty mieszadla : Inport  Port=6
  Booster : Product  RndMeth=Zero
  Booster block : Subsystem
  Constant : Constant  Value=0.2
  Divide : Product  Inputs=*/
  Dynamika rozkladu : Gain  Gain=1/100
  Ilosc : Integrator  LimitOutput=on  UpperSaturationLimit=48  LowerSaturationLimit=0
  Mieszadlo : DotProduct  OutDataTypeStr=Inherit: Inherit via internal rule
  Nasycenie : DotProduct  OutDataTypeStr=Inherit: Inherit via internal rule
  Odplyw srutu : DotProduct  OutDataTypeStr=Inherit: Inherit via internal rule
  Relational Operator1 : RelationalOperator  Operator=>  InputSameDT=off
  Sum : Sum  Inputs=|++
  Sum8 : Sum  Inputs=|+-
  Sum9 : Sum  Inputs=|+-
  Szybkosc reakcji : DotProduct  OutDataTypeStr=Inherit: Inherit via internal rule
  Warunki rozkladu : DotProduct  OutDataTypeStr=Inherit: Inherit via internal rule
  Wplyw mpieszadla : Gain  Gain=0.8/0.9563
  Wplyw temperatury : Lookup  InputValues=[0, 71, 74, 75, 76, 80, 100]  Table=[0, 0, 1, 1, 1, 0, 0]  SaturateOnIntegerOverflow=off
  Maltoza : Outport
  wires:
  Wplyw temperatury/1 -> Warunki rozkladu/2
  Ilosc/1 -> Sum8/2, Divide/1
  Szybkosc reakcji/1 -> Nasycenie/2
  Divide/1 -> Odplyw srutu/2, Relational Operator1/2, Maltoza/1
  Relational Operator1/1 -> Nasycenie/1
  Sum8/1 -> Szybkosc reakcji/2
  Sum9/1 -> Ilosc/1
  Nasycenie/1 -> Sum9/1
  Odplyw srutu/1 -> Sum9/2
  Srednia temperatura/1 -> Wplyw temperatury/1
  Objetosc mieszaniny/1 -> Divide/2, Sum8/1
  Odplyw/1 -> Odplyw srutu/1
  Jakosc mieszaniny/1 -> Warunki rozkladu/1
  Dekstryny/1 -> Relational Operator1/1
  Obroty mieszadla/1 -> Wplyw mpieszadla/1
  Wplyw mpieszadla/1 -> Sum/1
  Constant/1 -> Sum/2
  Sum/1 -> Mieszadlo/1
  Booster block/1(Out) -> Booster/2
  Mieszadlo/1 -> Dynamika rozkladu/1
  Warunki rozkladu/1 -> Mieszadlo/2
  Dynamika rozkladu/1 -> Booster/1
  Booster/1 -> Szybkosc reakcji/1

== system BrowarModel/Kadz zacierna/Kadz zacierna/Kadz zacierna/Model jakosci zacieru/Przerwa maltozowa ==
  note: Przerwa maltozowa
  Skrobia rozpuszczona : Inport
  Srednia temperatura : Inport  Port=2
  Jakosc mieszaniny : Inport  Port=3
  Objetosc mieszaniny : Inport  Port=4
  Odplyw : Inport  Port=5
  Obroty mieszadla : Inport  Port=6
  Booster : Product  RndMeth=Zero
  Booster block : Subsystem
  Constant : Constant  Value=0.2
  Divide : Product  Inputs=*/
  Dynamika rozkladu : Gain  Gain=1/100
  Ilosc : Integrator  LimitOutput=on  UpperSaturationLimit=48  LowerSaturationLimit=0
  Mieszadlo : DotProduct  OutDataTypeStr=Inherit: Inherit via internal rule
  Nasycenie : DotProduct  OutDataTypeStr=Inherit: Inherit via internal rule
  Odplyw srutu : DotProduct  OutDataTypeStr=Inherit: Inherit via internal rule
  Relational Operator1 : RelationalOperator  Operator=>  InputSameDT=off
  Sum : Sum  Inputs=|++
  Sum8 : Sum  Inputs=|+-
  Sum9 : Sum  Inputs=|+-
  Szybkosc reakcji : DotProduct  OutDataTypeStr=Inherit: Inherit via internal rule
  Warunki rozkladu : DotProduct  OutDataTypeStr=Inherit: Inherit via internal rule
  Wplyw mpieszadla : Gain  Gain=0.8/0.9563
  Wplyw temperatury : Lookup  InputValues=[0, 64, 67, 68, 69, 72, 100]  Table=[0, 0, 1, 1, 1, 0, 0]  SaturateOnIntegerOverflow=off
  Dekstryny : Outport
  wires:
  Jakosc mieszaniny/1 -> Warunki rozkladu/1
  Odplyw/1 -> Odplyw srutu/1
  Objetosc mieszaniny/1 -> Sum8/1, Divide/2
  Srednia temperatura/1 -> Wplyw temperatury/1
  Odplyw srutu/1 -> Sum9/2
  Nasycenie/1 -> Sum9/1
  Sum9/1 -> Ilosc/1
  Sum8/1 -> Szybkosc reakcji/2
  Relational Operator1/1 -> Nasycenie/1
  Divide/1 -> Relational Operator1/2, Odplyw srutu/2, Dekstryny/1
  Szybkosc reakcji/1 -> Nasycenie/2
  Ilosc/1 -> Sum8/2, Divide/1
  Wplyw temperatury/1 -> Warunki rozkladu/2
  Skrobia rozpuszczona/1 -> Relational Operator1/1
  Obroty mieszadla/1 -> Wplyw mpieszadla/1
  Wplyw mpieszadla/1 -> Sum/1
  Constant/1 -> Sum/2
  Sum/1 -> Mieszadlo/1
  Warunki rozkladu/1 -> Mieszadlo/2
  Mieszadlo/1 -> Dynamika rozkladu/1
  Booster/1 -> Szybkosc reakcji/1
  Dynamika rozkladu/1 -> Booster/1
  Booster block/1(Out) -> Booster/2

== system BrowarModel/Kadz zacierna/Kadz zacierna/Kadz zacierna/Model rozkladu temperatur/Gradient temperatury ==
  note: Gradient temperatury
  Poziom : Inport
  Temperatura otoczenia : Inport  Port=2
  Srednia temperatura : Inport  Port=3
  Obroty mieszadla : Inport  Port=4
  "  1/2  " : Gain  Gain=0.5
  " Dot  1" : DotProduct  OutDataTypeStr=Inherit: Inherit via internal rule
  " Gain 2" : Gain  Gain=2
  "1/2  " : Gain  Gain=0.5
  Fcn : Fcn  Expr=0.9*u(1)*(1-0.9*u(2))
  MinMax : MinMax
  Mux : Mux  Inputs=2
  Mux1 : Mux  Inputs=2
  Obroty skalowanie : Gain  Gain=1/2
  Poziom FS1 : Gain  Gain=1/2
  Sat : Saturate  UpperLimit=100  LowerLimit=0
  Sat doplyw Sat FS : Saturate  UpperLimit=1  LowerLimit=0
  Sat doplyw Sat FS1 : Saturate  UpperLimit=1  LowerLimit=0
  Saturation : Saturate  UpperLimit=100  LowerLimit=0
  Saturation1 : Saturate  UpperLimit=100  LowerLimit=0
  Sum1 : Sum  Inputs=|++
  Sum2 : Sum  Inputs=|-+
  Sum3 : Sum  Inputs=|+-
  Sum4 : Sum  Inputs=|-+
  Sum5 : Sum  Inputs=|++
  Sum7 : Sum  Inputs=|-+
  Sum8 : Sum  Inputs=|++
  Transfer Fcn : TransferFcn  Denominator=[10 1]
  Temperatura przy powierzchni : Outport
  Temperatura przy dnie : Outport  Port=2
  Gradient temperatury : Outport  Port=3
  wires:
  Fcn/1 -> Transfer Fcn/1
  Obroty skalowanie/1 -> Sat doplyw Sat FS/1  "FS"
  Obroty mieszadla/1 -> Obroty skalowanie/1  "obr/min"
  Poziom/1 -> Poziom FS1/1  "m"
  Sat doplyw Sat FS/1 -> Mux1/2
  Poziom FS1/1 -> Mux1/1
  Mux1/1 -> Fcn/1
  Sum8/1 -> Temperatura przy dnie/1
  " Gain 2"/1 -> Gradient temperatury/1
  Sum7/1 -> Temperatura przy powierzchni/1
  Temperatura otoczenia/1 -> Sum4/1
  Sat/1 -> " Gain 2"/1, Sum7/1, Sum8/1
  MinMax/1 -> Sat/1
  Mux/1 -> MinMax/1
  Sum3/1 -> Mux/2
  Sum5/1 -> Mux/1
  Saturation/1 -> Sum5/1
  Saturation1/1 -> Sum3/1
  Sum1/1 -> Saturation1/1
  Sum2/1 -> Saturation/1
  "  1/2  "/1 -> Sum2/1
  "1/2  "/1 -> Sum1/1
  " Dot  1"/1 -> "  1/2  "/1, "1/2  "/1
  Sum4/1 -> " Dot  1"/2
  Sat doplyw Sat FS1/1 -> " Dot  1"/1
  Transfer Fcn/1 -> Sat doplyw Sat FS1/1
  Srednia temperatura/1 -> Sum7/2, Sum5/2, Sum3/2, Sum2/2, Sum1/2, Sum4/2, Sum8/2

== system BrowarModel/Mlyn browarniany/Mlyn browarniany/Dozownik mlyna/Dozownik turbinowy/Zaklocenia ==
  note: Zaklocenia procesowe
  In : Inport
  Product3 : Product  InputSameDT=on  RndMeth=Zero  SaturateOnIntegerOverflow=on  OutDataTypeStr=Inherit: Same as first input
  Product4 : Product  InputSameDT=on  RndMeth=Zero  SaturateOnIntegerOverflow=on  OutDataTypeStr=Inherit: Same as first input
  Random Number : RandomNumber  Variance=0.1  Seed=4365624  SampleTime=0.1
  Transfer Fcn1 : TransferFcn  Denominator=[1 1]
  Out : Outport
  wires:
  [ZaklProc] -> Product3/2
  Random Number/1 -> Product3/1
  Product3/1 -> Transfer Fcn1/1
  Transfer Fcn1/1 -> Product4/2
  In/1 -> Product4/1
  Product4/1 -> Out/1

== system BrowarModel/Mlyn browarniany/Mlyn browarniany/Dozownik mlyna/Silnik elektryczny/Stan ==
  Zalaczony : Inport
  Zdatny : Inport  Port=2
  Add : Sum  Inputs=+++
  Alarm1 : Logic  Operator=NOT  AllPortsSameDT=off
  Alarm2 : Gain  Gain=3
  Display : Display
  GUIMon : Gain
  Idle1 : Logic  AllPortsSameDT=off
  Idle2 : Logic  Operator=NOT  AllPortsSameDT=off
  Idle3 : Gain
  Running1 : Logic  AllPortsSameDT=off
  Running2 : Gain  Gain=2
  Idle : Outport
  Running : Outport  Port=2
  Alarm : Outport  Port=3
  wires:
  Running1/1 -> Running/1, Running2/1
  Idle1/1 -> Idle/1, Idle3/1
  Zalaczony/1 -> Running1/1, Idle2/1
  Zdatny/1 -> Alarm1/1, Running1/2, Idle1/2
  Alarm1/1 -> Alarm/1, Alarm2/1
  Idle2/1 -> Idle1/1
  Idle3/1 -> Add/1
  Running2/1 -> Add/2
  Alarm2/1 -> Add/3
  Add/1 -> GUIMon/1
  GUIMon/1 -> Display/1

== system BrowarModel/Mlyn browarniany/Mlyn browarniany/Dozownik mlyna/Silnik elektryczny/Sterowanie ==
  note: Sterowanie silnika elektrycznego
  Zadane obroty : Inport
  Zalaczenie : Inport  Port=2
  Hz : Gain  Gain=45/100
  Min sterowanie : Constant  Value=5
  Relay : Relay
  Saturation [0,100] : Saturate  UpperLimit=100  LowerLimit=0
  "Sterowanie " : DotProduct  OutDataTypeStr=Inherit: Inherit via internal rule
  Sum2 : Sum  Inputs=|++
  Sterowanie : Outport
  wires:
  Relay/1 -> "Sterowanie "/1  "{0,1}"
  Saturation [0,100]/1 -> Hz/1
  Hz/1 -> Sum2/1  "Hz"
  Min sterowanie/1 -> Sum2/2  "Hz"
  Sum2/1 -> "Sterowanie "/2
  Zalaczenie/1 -> Relay/1  "{0,1}"
  "Sterowanie "/1 -> Sterowanie/1  "Hz"
  Zadane obroty/1 -> Saturation [0,100]/1  "[0,100]"

== system BrowarModel/Mlyn browarniany/Mlyn browarniany/Dozownik mlyna/Silnik elektryczny/Sterownik ==
  PV : Inport
  SP : Inport  Port=2
  Integrator : Integrator  LimitOutput=on  UpperSaturationLimit=50  LowerSaturationLimit=0
  K : Gain
  Saturation [0,50] : Saturate  UpperLimit=50  LowerLimit=0
  Sum2 : Sum  Inputs=|+-
  Sum3 : Sum  Inputs=|++
  Ti : Gain
  CV : Outport
  wires:
  Sum2/1 -> K/1
  Integrator/1 -> Sum3/1
  K/1 -> Ti/1, Sum3/2
  Ti/1 -> Integrator/1
  PV/1 -> Sum2/2
  SP/1 -> Sum2/1
  Sum3/1 -> Saturation [0,50]/1
  Saturation [0,50]/1 -> CV/1

== system BrowarModel/Mlyn browarniany/Mlyn browarniany/Dozownik mlyna/Silnik elektryczny/Zaklocenia ==
  note: Zaklocenia procesowe
  In : Inport
  Product3 : Product  InputSameDT=on  RndMeth=Zero  SaturateOnIntegerOverflow=on  OutDataTypeStr=Inherit: Same as first input
  Product4 : Product  InputSameDT=on  RndMeth=Zero  SaturateOnIntegerOverflow=on  OutDataTypeStr=Inherit: Same as first input
  Random Number : RandomNumber  Variance=0.05  Seed=4365624  SampleTime=0.1
  Transfer Fcn1 : TransferFcn  Denominator=[1 1]
  Transfer Fcn2 : TransferFcn  Denominator=[1 1]
  Transfer Fcn3 : TransferFcn  Denominator=[1 1]
  Out : Outport
  wires:
  [ZaklProc] -> Product3/2
  Random Number/1 -> Product3/1
  Product3/1 -> Transfer Fcn1/1
  Transfer Fcn1/1 -> Transfer Fcn2/1
  In/1 -> Product4/1
  Product4/1 -> Out/1
  Transfer Fcn2/1 -> Transfer Fcn3/1
  Transfer Fcn3/1 -> Product4/2

== system BrowarModel/Mlyn browarniany/Mlyn browarniany/Walce mlyna/Komora nad walcami/Detektory poziomu ==
  note: Detektory poziomu
  Poziom : Inport
  Pozycja sensora max : Constant  Value=0.7
  Pozycja sensora min : Constant  Value=0.3
  Sensor max : RelationalOperator  InputSameDT=off
  Sensor min : RelationalOperator  InputSameDT=off
  Poziom  wysoki : Outport
  Poziom niski : Outport  Port=2
  wires:
  Sensor min/1 -> Poziom niski/1
  Sensor max/1 -> Poziom  wysoki/1
  Pozycja sensora min/1 -> Sensor min/2
  Pozycja sensora max/1 -> Sensor max/2
  Poziom/1 -> Sensor max/1, Sensor min/1  "m"

== system BrowarModel/Mlyn browarniany/Mlyn browarniany/Walce mlyna/Silnik elektryczny/Stan ==
  Zalaczony : Inport
  Zdatny : Inport  Port=2
  Add : Sum  Inputs=+++
  Alarm1 : Logic  Operator=NOT  AllPortsSameDT=off
  Alarm2 : Gain  Gain=3
  Display : Display
  GUIMon : Gain
  Idle1 : Logic  AllPortsSameDT=off
  Idle2 : Logic  Operator=NOT  AllPortsSameDT=off
  Idle3 : Gain
  Running1 : Logic  AllPortsSameDT=off
  Running2 : Gain  Gain=2
  Idle : Outport
  Running : Outport  Port=2
  Alarm : Outport  Port=3
  wires:
  Running1/1 -> Running/1, Running2/1
  Idle1/1 -> Idle/1, Idle3/1
  Zalaczony/1 -> Running1/1, Idle2/1
  Zdatny/1 -> Alarm1/1, Running1/2, Idle1/2
  Alarm1/1 -> Alarm/1, Alarm2/1
  Idle2/1 -> Idle1/1
  Idle3/1 -> Add/1
  Running2/1 -> Add/2
  Alarm2/1 -> Add/3
  Add/1 -> GUIMon/1
  GUIMon/1 -> Display/1

== system BrowarModel/Mlyn browarniany/Mlyn browarniany/Walce mlyna/Silnik elektryczny/Sterowanie ==
  note: Sterowanie silnika elektrycznego
  Zadane obroty : Inport
  Zalaczenie : Inport  Port=2
  Hz : Gain  Gain=45/100
  Min sterowanie : Constant  Value=5
  Relay : Relay
  Saturation [0,100] : Saturate  UpperLimit=100  LowerLimit=0
  "Sterowanie " : DotProduct  OutDataTypeStr=Inherit: Inherit via internal rule
  Sum2 : Sum  Inputs=|++
  Sterowanie : Outport
  wires:
  Relay/1 -> "Sterowanie "/1  "{0,1}"
  Saturation [0,100]/1 -> Hz/1
  Hz/1 -> Sum2/1  "Hz"
  Min sterowanie/1 -> Sum2/2  "Hz"
  Sum2/1 -> "Sterowanie "/2
  Zalaczenie/1 -> Relay/1  "{0,1}"
  "Sterowanie "/1 -> Sterowanie/1  "Hz"
  Zadane obroty/1 -> Saturation [0,100]/1  "[0,100]"

== system BrowarModel/Mlyn browarniany/Mlyn browarniany/Walce mlyna/Silnik elektryczny/Sterownik ==
  PV : Inport
  SP : Inport  Port=2
  Integrator : Integrator  LimitOutput=on  UpperSaturationLimit=50  LowerSaturationLimit=0
  K : Gain
  Saturation [0,50] : Saturate  UpperLimit=50  LowerLimit=0
  Sum2 : Sum  Inputs=|+-
  Sum3 : Sum  Inputs=|++
  Ti : Gain
  CV : Outport
  wires:
  Sum2/1 -> K/1
  Integrator/1 -> Sum3/1
  K/1 -> Ti/1, Sum3/2
  Ti/1 -> Integrator/1
  PV/1 -> Sum2/2
  SP/1 -> Sum2/1
  Sum3/1 -> Saturation [0,50]/1
  Saturation [0,50]/1 -> CV/1

== system BrowarModel/Mlyn browarniany/Mlyn browarniany/Walce mlyna/Silnik elektryczny/Zaklocenia ==
  note: Zaklocenia procesowe
  In : Inport
  Product3 : Product  InputSameDT=on  RndMeth=Zero  SaturateOnIntegerOverflow=on  OutDataTypeStr=Inherit: Same as first input
  Product4 : Product  InputSameDT=on  RndMeth=Zero  SaturateOnIntegerOverflow=on  OutDataTypeStr=Inherit: Same as first input
  Random Number : RandomNumber  Variance=0.05  Seed=4365624  SampleTime=0.1
  Transfer Fcn1 : TransferFcn  Denominator=[1 1]
  Transfer Fcn2 : TransferFcn  Denominator=[1 1]
  Transfer Fcn3 : TransferFcn  Denominator=[1 1]
  Out : Outport
  wires:
  [ZaklProc] -> Product3/2
  Random Number/1 -> Product3/1
  Product3/1 -> Transfer Fcn1/1
  Transfer Fcn1/1 -> Transfer Fcn2/1
  In/1 -> Product4/1
  Product4/1 -> Out/1
  Transfer Fcn2/1 -> Transfer Fcn3/1
  Transfer Fcn3/1 -> Product4/2

== system BrowarModel/Mlyn browarniany/Mlyn browarniany/Walce mlyna/Walce/Zaklocenia ==
  note: Zaklocenia procesowe
  In : Inport
  Product3 : Product  InputSameDT=on  RndMeth=Zero  SaturateOnIntegerOverflow=on  OutDataTypeStr=Inherit: Same as first input
  Product4 : Product  InputSameDT=on  RndMeth=Zero  SaturateOnIntegerOverflow=on  OutDataTypeStr=Inherit: Same as first input
  Random Number : RandomNumber  Variance=0.1  Seed=4365624  SampleTime=0.1
  Transfer Fcn1 : TransferFcn  Denominator=[1 1]
  Out : Outport
  wires:
  [ZaklProc] -> Product3/2
  Random Number/1 -> Product3/1
  Product3/1 -> Transfer Fcn1/1
  Transfer Fcn1/1 -> Product4/2
  In/1 -> Product4/1
  Product4/1 -> Out/1

== system BrowarModel/Kadz zacierna/Kadz zacierna/Kadz zacierna/Model jakosci zacieru/Przerwa bialkowa /Booster block ==
  Fast : Constant  Value=2
  Normal : Constant
  Switch : Switch  Threshold=0.5  SaturateOnIntegerOverflow=off  InputSameDT=off
  Out : Outport
  wires:
  [TrybSym] -> Switch/2
  Fast/1 -> Switch/1
  Normal/1 -> Switch/3
  Switch/1 -> Out/1

== system BrowarModel/Kadz zacierna/Kadz zacierna/Kadz zacierna/Model jakosci zacieru/Przerwa dekstrynujaca/Booster block ==
  Fast : Constant  Value=2
  Normal : Constant
  Switch : Switch  Threshold=0.5  SaturateOnIntegerOverflow=off  InputSameDT=off
  Out : Outport
  wires:
  [TrybSym] -> Switch/2
  Fast/1 -> Switch/1
  Normal/1 -> Switch/3
  Switch/1 -> Out/1

== system BrowarModel/Kadz zacierna/Kadz zacierna/Kadz zacierna/Model jakosci zacieru/Przerwa maltozowa/Booster block ==
  Fast : Constant  Value=2
  Normal : Constant
  Switch : Switch  Threshold=0.5  SaturateOnIntegerOverflow=off  InputSameDT=off
  Out : Outport
  wires:
  [TrybSym] -> Switch/2
  Fast/1 -> Switch/1
  Normal/1 -> Switch/3
  Switch/1 -> Out/1
